simulink model "SeperatelyExcited"  (R2019a)
settings: Solver=VariableStepAuto  StartTime=0.0  StopTime=10.0  RelTol=1e-3
InitFcn:
  | run MotorParameter_Initialize
undefined symbols (not defined in the file): Bm, J, Laa, Laf, Lff, Ra, Rf
settings Model: Creator=visha  LastModifiedBy=visha

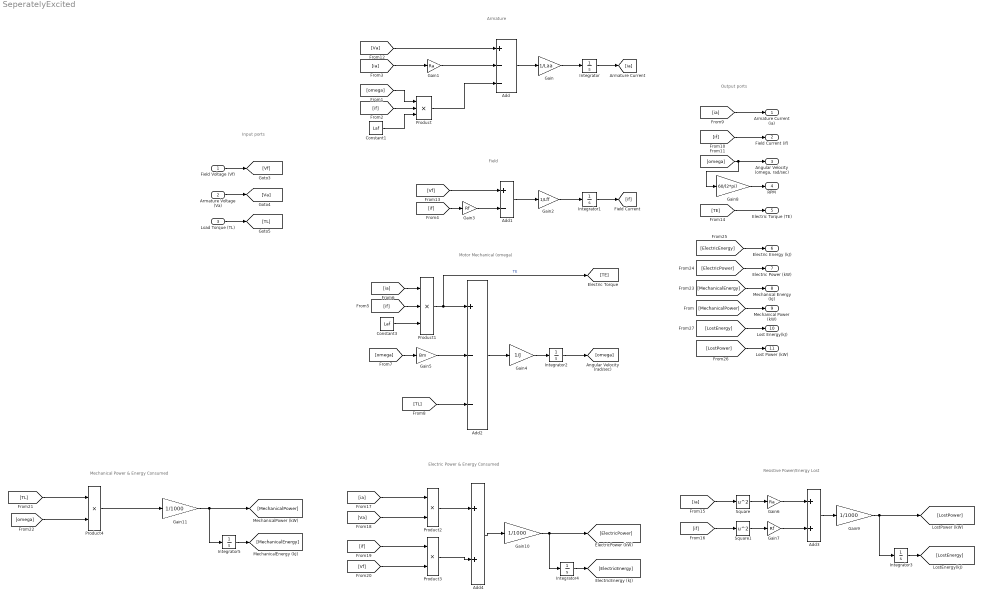
== system SeperatelyExcited ==
  note: Field
  note: Armature
  note: Motor Mechanical (omega)
  note: Output ports
  note: Input ports
  note: Resistive Power/Energy Lost
  note: Electric Power & Energy Consumed
  note: Mechanical Power & Energy Consumed
  Field Voltage (Vf) : Inport
  Armature Voltage (Va) : Inport  Port=2
  Load Torque (TL) : Inport  Port=3
  Add : Sum  Inputs=+--
  Add1 : Sum  Inputs=+-
  Add2 : Sum  Inputs=+--
  Add3 : Sum
  Add4 : Sum
  Constant1 : Constant  Value=Laf
  Constant3 : Constant  Value=Laf
  Gain : Gain  Gain=1/Laa
  Gain1 : Gain  Gain=Ra
  Gain10 : Gain  Gain=1/1000
  Gain11 : Gain  Gain=1/1000
  Gain2 : Gain  Gain=1/Lff
  Gain3 : Gain  Gain=Rf
  Gain4 : Gain  Gain=1/J
  Gain5 : Gain  Gain=Bm
  Gain6 : Gain  Gain=Ra
  Gain7 : Gain  Gain=Rf
  Gain8 : Gain  Gain=60/(2*pi)
  Gain9 : Gain  Gain=1/1000
  Integrator{,1..5} (6 alike) : Integrator
  Product : Product  Inputs=3
  Product1 : Product  Inputs=3
  Product2 : Product
  Product3 : Product
  Product4 : Product
  Square : Math  Operator=square  SaturateOnIntegerOverflow=on
  Square1 : Math  Operator=square  SaturateOnIntegerOverflow=on
  Armature Current (ia) : Outport
  Field Current (if) : Outport  Port=2
  "Angular Velocity (omega, rad/sec)" : Outport  Port=3
  RPM : Outport  Port=4
  Electric Torque (TE) : Outport  Port=5
  Electric Energy (kJ) : Outport  Port=6
  Electric Power (kW) : Outport  Port=7
  Mechanical Energy (kJ) : Outport  Port=8
  Mechanical Power (kW) : Outport  Port=9
  Lost Energy(kJ) : Outport  Port=10
  Lost Power (kW) : Outport  Port=11
  wires:
  Gain/1 -> Integrator/1
  Add/1 -> Gain/1
  Integrator/1 -> [ia]
  [ia] -> Gain1/1
  Gain1/1 -> Add/2
  [if] -> Product/2
  [omega] -> Product/1
  Constant1/1 -> Product/3
  Product/1 -> Add/3
  Integrator1/1 -> [if]
  Gain2/1 -> Integrator1/1
  Gain3/1 -> Add1/2
  [Vf] -> Add1/1
  [if] -> Gain3/1
  Add1/1 -> Gain2/1
  [ia] -> Product1/1
  [if] -> Product1/2
  Constant3/1 -> Product1/3
  Add2/1 -> Gain4/1
  Product1/1 -> [TE], Add2/1  "TE"
  Gain4/1 -> Integrator2/1
  Integrator2/1 -> [omega]
  Gain5/1 -> Add2/2
  [TL] -> Add2/3
  [ia] -> Armature Current (ia)/1
  [if] -> Field Current (if)/1
  [omega] -> Gain8/1, "Angular Velocity (omega, rad/sec)"/1
  [Va] -> Add/1
  Field Voltage (Vf)/1 -> [Vf]
  Armature Voltage (Va)/1 -> [Va]
  Load Torque (TL)/1 -> [TL]
  [TE] -> Electric Torque (TE)/1
  [ia] -> Square/1
  [if] -> Square1/1
  Square1/1 -> Gain7/1
  Square/1 -> Gain6/1
  Gain7/1 -> Add3/2
  Gain6/1 -> Add3/1
  Add3/1 -> Gain9/1
  Integrator3/1 -> [LostEnergy]
  [ia] -> Product2/1
  [Va] -> Product2/2
  Product2/1 -> Add4/1
  Product3/1 -> Add4/2
  [Vf] -> Product3/2
  [if] -> Product3/1
  Add4/1 -> Gain10/1
  Gain8/1 -> RPM/1
  Gain9/1 -> [LostPower], Integrator3/1
  Integrator4/1 -> [ElectricEnergy]
  Gain10/1 -> [ElectricPower], Integrator4/1
  [omega] -> Product4/2
  [TL] -> Product4/1
  Product4/1 -> Gain11/1
  Gain11/1 -> Integrator5/1, [MechanicalPower]
  Integrator5/1 -> [MechanicalEnergy]
  [ElectricEnergy] -> Electric Energy (kJ)/1
  [ElectricPower] -> Electric Power (kW)/1
  [MechanicalEnergy] -> Mechanical Energy (kJ)/1
  [MechanicalPower] -> Mechanical Power (kW)/1
  [LostEnergy] -> Lost Energy(kJ)/1
  [LostPower] -> Lost Power (kW)/1
  [omega] -> Gain5/1
